simulink model "torque_vectoring"  (R2023b)
settings: Solver=FixedStepDiscrete  StartTime=0.0  StopTime=3180  FixedStep=0.015  RelTol=1e-3
settings Model: TunableVars=Ib,ub,Tmc,Tmo,k_TL,dIb,I_FUSE,PLb,r_power_sat,yaw_table,v,s,half_track  TunableVarsStorageClass=Auto,Auto,Auto,Auto,Auto,Auto,Auto,Auto,Auto,Auto,Auto,Auto,Auto  TunableVarsTypeQualifier=,,,,,,,,,,,,  Creator=Inver  LastModifiedBy=Inver
settings DataIOCC: ExternalInput=ds_tv.getElement('R'),ds_tv.getElement('F_raw'),ds_tv.getElement('D_raw'),ds_tv.getElement('dphi'),ds_tv.getElement('TVS_P'),ds_tv.getElement('TVS_I')  LoadExternalInput=on
settings OptimizationCC: DefaultParameterBehavior=Inlined  GainParamInheritBuiltInType=on  UseFloatMulNetSlope=on  UseSpecifiedMinMax=on  InlineInvariantSignals=on  StrengthReduction=on  PassReuseOutputArgsAs=Individual arguments  ZeroExternalMemoryAtStartup=off  ZeroInternalMemoryAtStartup=off  NoFixptDivByZeroProtection=on  EfficientFloat2IntCast=on  LifeSpan=1  OptimizeBlockOrder=speed  DifferentSizesBufferReuse=on  OptimizationPriority=Speed  MultiThreadedLoops=on  EfficientTunableParamExpr=on
settings DebuggingCC: ParameterTunabilityLossMsg=error
settings HardwareCC: ProdBitPerPointer=32  ProdBitPerSizeT=32  ProdBitPerPtrDiffT=32  ProdLargestAtomicInteger=Long  ProdLargestAtomicFloat=Double  ProdWordSize=32  ProdLongLongMode=on  ProdHWDeviceType=ARM Compatible->ARM Cortex-M
settings SFSimCC: MATLABDynamicMemAlloc=off
settings RTWCC: Description=Embedded Coder  SystemTargetFile=ert.tlc  GenCodeOnly=on  PackageGeneratedCodeAndArtifacts=on  TemplateMakefile=ert_default_tmf  Toolchain=GNU Tools for ARM Embedded Processors  BuildConfiguration=Faster Runs  CheckMdlBeforeBuild=Warning
settings CodeAppCC: ForceParamTrailComments=on  IgnoreCustomStorageClasses=off  SimulinkDataObjDesc=on  SimulinkBlockComments=off
settings ERTTargetCC: TargetLangStandard=C99 (ISO)  GenerateSampleERTMain=on  CombineSignalStateStructs=on  SuppressErrorStatus=on  SupportNonFinite=off  SupportComplex=off  InlinedParameterPlacement=NonHierarchical  ERTCustomFileTemplate=example_file_process.tlc  GlobalDataDefinition=InSeparateSourceFile  DataDefinitionFile=data.c  GlobalDataReference=InSeparateHeaderFile  ERTFilePackagingFormat=CompactWithDataFile  DataReferenceFile=data.h

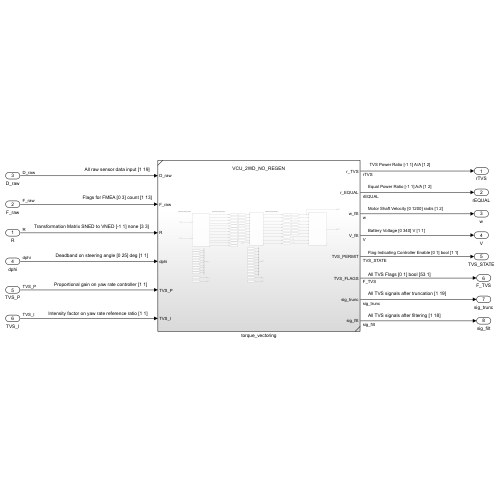
[thumbnail: Simulink's stored preview of the top-level diagram]
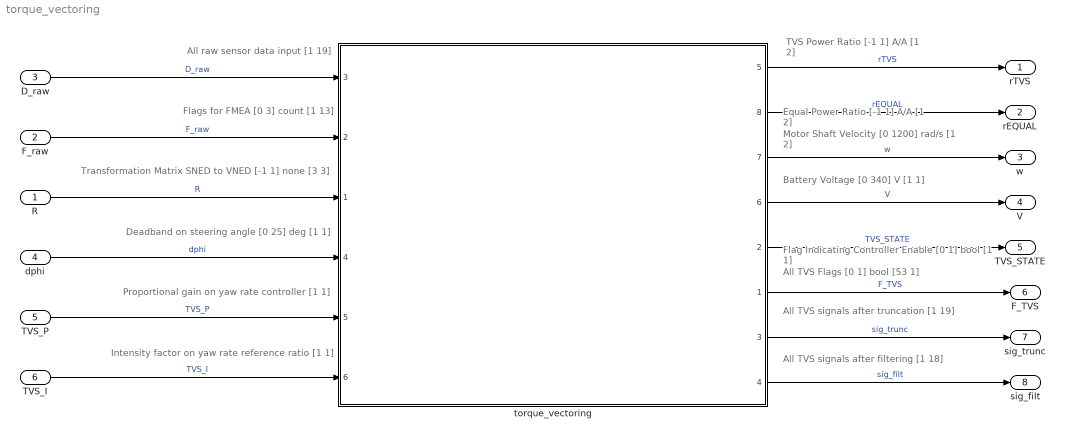
== system torque_vectoring ==
  note: All TVS signals after truncation [1 19]
  note: All TVS Flags [0 1] bool [53 1]
  note: Transformation Matrix SNED to VNED [-1 1] none [3 3]
  note: Proportional gain on yaw rate controller [1 1]
  note: Intensity factor on yaw rate reference ratio [1 1]
  note: Deadband on steering angle [0 25] deg [1 1]
  note: All raw sensor data input [1 19]
  note: Flags for FMEA [0 3] count [1 13]
  note: Battery Voltage [0 340] V [1 1]
  note: TVS Power Ratio [-1 1] A/A [1 2]
  note: Motor Shaft Velocity [0 1200] rad/s [1 2]
  note: Equal Power Ratio [-1 1] A/A [1 2]
  note: Flag Indicating Controller Enable [0 1] bool [1 1]
  note: All TVS signals after filtering [1 18]
  R : Inport  PortDimensions=[3 3]
  F_raw : Inport  Port=2  PortDimensions=13
  D_raw : Inport  Port=3  PortDimensions=19
  dphi : Inport  Port=4  PortDimensions=1
  TVS_P : Inport  Port=5  PortDimensions=1
  TVS_I : Inport  Port=6  PortDimensions=1
  torque_vectoring : Subsystem  ReferencedSubsystem=VCU_2WD_NO_REGEN
      settings: PortSchema="{\"entries\":[{\"content\":{\"sides\":[{\"content\":{\"connectorIds\":[\"In3\",\"In2\",\"In1\",\"In4\",\"In5\",\"In6\"]},\"type\":\"ConnectorPlacement.EquallySpacedRectSide\",\"uuid\":\"3c8e8a37-ef6f-4083-861d-4f5221941564\"},{\"content\":{\"connectorIds\":[\"Out5\",\"Out8\",\"Out7\",\"Out6\",\"Out2\",\"Out1\",\"Out3\",\"Out4\"],\"side\":\"RIGHT\"},\"type\":\"ConnectorPlacement.EquallySpacedRectSide\",\"uuid\":\"6ecab03b-b901-45ae-96b7-b90ac27ccb5d\"},{\"content\":{\"side\":\"TOP\"},\"type\":\"ConnectorPlacement.EquallySpacedRectSide\",\"uuid\":\"873f5b8f-9412-4a99-9fa6-4198568ce17c\"}]},\"type\":\"ConnectorPlacement.EquallySpacedConnector\",\"uuid\":\"f40c1818-feda-414e-9f19-b565b0263b38\"}],\"packageUris\":[\"http://schema.mathworks.com/mf0/Connector/R2020b\"],\"version\":\"1.0\"}"
  rTVS : Outport
  rEQUAL : Outport  Port=2
  w : Outport  Port=3
  V : Outport  Port=4
  TVS_STATE : Outport  Port=5
  F_TVS : Outport  Port=6
  sig_trunc : Outport  Port=7
  sig_filt : Outport  Port=8
  wires:
  torque_vectoring/7 -> w/1  "w"
  torque_vectoring/2 -> TVS_STATE/1  "TVS_STATE"
  torque_vectoring/4 -> sig_filt/1  "sig_filt"
  torque_vectoring/6 -> V/1  "V"
  torque_vectoring/8 -> rEQUAL/1  "rEQUAL"
  torque_vectoring/1 -> F_TVS/1  "F_TVS"
  torque_vectoring/5 -> rTVS/1  "rTVS"
  torque_vectoring/3 -> sig_trunc/1  "sig_trunc"
  R/1 -> torque_vectoring/1  "R"
  F_raw/1 -> torque_vectoring/2  "F_raw"
  D_raw/1 -> torque_vectoring/3  "D_raw"
  dphi/1 -> torque_vectoring/4  "dphi"
  TVS_P/1 -> torque_vectoring/5  "TVS_P"
  TVS_I/1 -> torque_vectoring/6  "TVS_I"
